simulink model "q1"  (Simulink 7.1)
settings: Solver=ode45  StartTime=0.0  StopTime=100  RelTol=1e-3
values from neighbouring files (symbols this model uses):
  A = [-((1/RC)*(2 - K)) ((1/RC)*K)  -(1/RC) ... (first row only)    [script.m]
  B = [(1/RC)*(2 - K); -(1/RC)*K; -(1/RC)*K]    [script.m]
  C_ = [C ... (first row only)    [script.m]
  D_ = [D; 0 ; 0 ; 0]    [script.m]
  X01 = [10; 10; 15]    [script.m]
  X02 = [10; -10; -10]    [script.m]
settings Model: Creator=ALUNO  LastModifiedBy=ALUNO

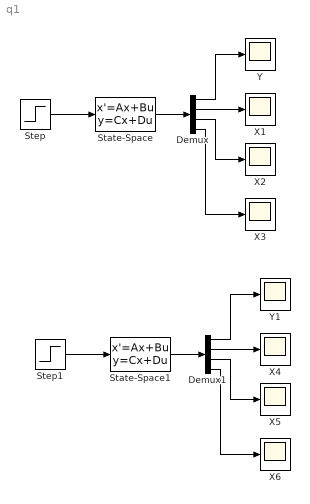
== system q1 ==
  Demux : Demux
  Demux1 : Demux
  State-Space : StateSpace  A=A  B=B  C=C_  D=D_  X0=X01
  State-Space1 : StateSpace  A=A  B=B  C=C_  D=D_  X0=X02
  Step : Step  Time=0  After=0  SampleTime=0
  Step1 : Step  Time=0  After=0  SampleTime=0
  X{1..6} (6 alike) : Scope
      X1 settings: YMin=1.39  YMax=1.61
      X2 settings: YMin=1.39  YMax=1.61  SaveName=ScopeData2
      X3 settings: YMin=1.39  YMax=1.61  SaveName=ScopeData3
      X4 settings: YMin=1.39  YMax=1.61  SaveName=ScopeData4
      X5 settings: YMin=1.39  YMax=1.61  SaveName=ScopeData5
      X6 settings: YMin=1.39  YMax=1.61  SaveName=ScopeData6
  Y : Scope
      settings: YMin=1.39  YMax=1.61
  Y1 : Scope
      settings: YMin=1.39  YMax=1.61  SaveName=ScopeData7
  wires:
  Step/1 -> State-Space/1
  State-Space/1 -> Demux/1
  Demux/1 -> Y/1
  Demux/2 -> X1/1
  Demux/3 -> X2/1
  Demux/4 -> X3/1
  Step1/1 -> State-Space1/1
  State-Space1/1 -> Demux1/1
  Demux1/1 -> Y1/1
  Demux1/2 -> X4/1
  Demux1/3 -> X5/1
  Demux1/4 -> X6/1
